simulink model "simSLIPModel"  (R2015a)
settings: Solver=ode45  StartTime=0.0  StopTime=2  FixedStep=0.001  RelTol=1e-6
values from neighbouring files (symbols this model uses):
  kIn = 50    [exhaustive.m]    (also in funkyFunc.m; heightConstraint.m; simVis.m)
  qIn = [q(1); q(2); dti; dri]    [exhaustive.m]    (also in funkyFunc.m; heightConstraint.m; simVis.m = [Thf0(1); Thf0(2); dti; dri])
  r0 = sym('r0', [noLinks 1])    [Generalised_SLIP_Model.m]    (also in Generalised_SLIP_Model_flight.m; exhaustive.m = 2; exhaustiveSearch.m = 2; funkyFunc.m = 2)
undefined symbols (not defined in the file or in its folder): k1, k2, k3, k4, k5
libraries: simulink x3, dspsigops x1
settings Model: Creator=STNNEI001  LastModifiedBy=STNNEI001
settings SolverCC: ZeroCrossAlgorithm=Adaptive
settings DataIOCC: ExternalInput=[qIn]  ReturnWorkspaceOutputs=on
settings DebuggingCC: UnderspecifiedInitializationDetection=Classic  MergeDetectMultiDrivingBlocksExec=none  MaxConsecutiveZCsMsg=none  MaskedZcDiagnostic=none  SolverPrmCheckMsg=warning  StateNameClashWarn=warning

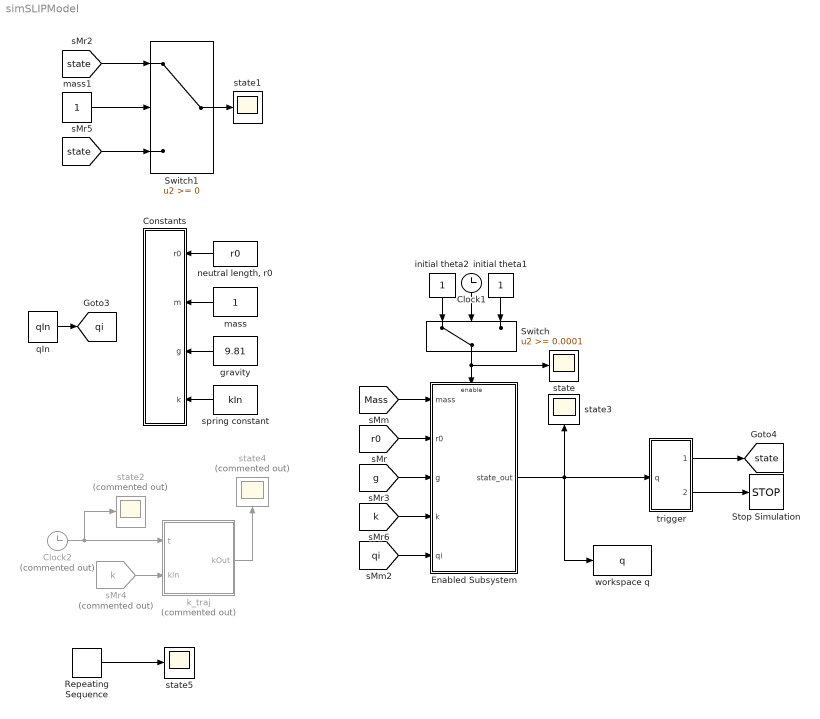
== system simSLIPModel ==
  Clock1 : Clock
  Clock2 : Clock  Commented=on
  Constants : Subsystem
  Enabled Subsystem : Subsystem  TreatAsAtomicUnit=on
  Repeating Sequence : simulink/Sources/Repeating Sequence  rep_seq_t=[0 0.05 0.1 0.15 0.32]  rep_seq_y=[k1 k2 k3 k4 k5]
  Stop Simulation : Stop
  Switch : Switch  Threshold=0.0001
  Switch1 : Switch
  gravity : Constant  Value=9.81
  initial theta1 : Constant
  initial theta2 : Constant
  k_traj : MATLAB Function  Commented=on  TreatAsAtomicUnit=on
  mass : Constant
  mass1 : Constant
  "neutral length, r0" : Constant  Value=r0
  qIn : Constant  Value=qIn
  sMr4 : From  Commented=on  GotoTag=k  TagVisibility=global
  spring constant : Constant  Value=kIn  VectorParams1D=off
  state{,1,3,5} (4 alike) : Scope
      state settings: SaveName=ScopeData16
      state1 settings: SaveName=ScopeData3
      state3 settings: SaveName=ScopeData15
      state5 settings: SaveName=ScopeData12
  state2 : Scope  Commented=on
      settings: SaveName=ScopeData4
  state4 : Scope  Commented=on
      settings: SaveName=ScopeData5
  trigger : Subsystem
  workspace q : ToWorkspace  VariableName=q  SaveFormat=Structure With Time  SampleTime=0.01
  tag scope: qi=global, state=global
  wires:
  "neutral length, r0"/1 -> Constants/1(r0)
  mass/1 -> Constants/2(m)
  gravity/1 -> Constants/3(g)
  spring constant/1 -> Constants/4(k)
  [Mass] -> Enabled Subsystem/1(mass)
  [r0] -> Enabled Subsystem/2(r0)
  [g] -> Enabled Subsystem/3(g)
  [qi] -> Enabled Subsystem/5(qi)
  Switch/1 -> state/1, Enabled Subsystem/Enable
  trigger/1(state) -> [state]
  Clock1/1 -> Switch/2
  initial theta1/1 -> Switch/3
  initial theta2/1 -> Switch/1
  Enabled Subsystem/1(state_out) -> trigger/1(q), workspace q/1, state3/1
  Switch1/1 -> state1/1
  [state] -> Switch1/1
  qIn/1 -> [qi]
  [state] -> Switch1/3
  sMr4/1 -> k_traj/2(kIn)
  Clock2/1 -> state2/1, k_traj/1(t)
  k_traj/1(kOut) -> state4/1
  [k] -> Enabled Subsystem/4(k)
  trigger/2(stop) -> Stop Simulation/1
  mass1/1 -> Switch1/2
  Repeating Sequence/1 -> state5/1

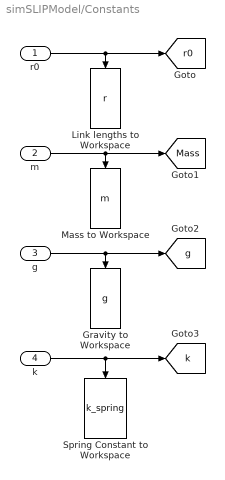
== system simSLIPModel/Constants ==
  r0 : Inport
  m : Inport  Port=2
  g : Inport  Port=3
  k : Inport  Port=4
  Gravity to Workspace : ToWorkspace  VariableName=g  SampleTime=-1
      settings: MaxDataPoints=1
  Link lengths to Workspace : ToWorkspace  VariableName=r  SampleTime=-1
      settings: MaxDataPoints=1
  Mass to Workspace : ToWorkspace  VariableName=m  SampleTime=-1
      settings: MaxDataPoints=1
  Spring Constant to Workspace : ToWorkspace  VariableName=k_spring  SampleTime=-1
      settings: MaxDataPoints=1
  tag scope: Mass=global, g=global, k=global, r0=global
  wires:
  m/1 -> [Mass], Mass to Workspace/1
  r0/1 -> Link lengths to Workspace/1, [r0]
  g/1 -> [g], Gravity to Workspace/1
  k/1 -> [k], Spring Constant to Workspace/1

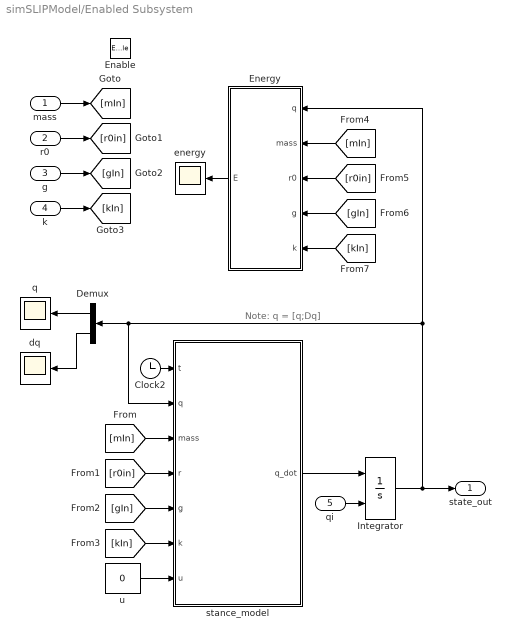
== system simSLIPModel/Enabled Subsystem ==
  note: Note: q = [q;Dq]
  mass : Inport
  r0 : Inport  Port=2
  g : Inport  Port=3
  k : Inport  Port=4
  qi : Inport  Port=5
  Enable : EnablePort
  Clock2 : Clock
  Demux : Demux  Outputs=2
  "Energy " : MATLAB Function  TreatAsAtomicUnit=on
  Integrator : Integrator  InitialConditionSource=external  InitialCondition=[pi/2;1;0;0]
  dq : Scope
      settings: SaveName=ScopeData7
  energy : Scope
  q : Scope
      settings: SaveName=ScopeData6
  stance_model : MATLAB Function  TreatAsAtomicUnit=on
  u : Constant  Value=0
  state_out : Outport
  wires:
  stance_model/1(q_dot) -> Integrator/1
  Integrator/1 -> state_out/1, stance_model/2(q), Demux/1, "Energy "/1(q)
  Demux/1 -> q/1
  Demux/2 -> dq/1
  [r0in] -> stance_model/4(r)
  [mIn] -> stance_model/3(mass)
  [gIn] -> stance_model/5(g)
  [kIn] -> stance_model/6(k)
  "Energy "/1(E) -> energy/1
  qi/1 -> Integrator/2
  u/1 -> stance_model/7(u)
  k/1 -> [kIn]
  g/1 -> [gIn]
  r0/1 -> [r0in]
  mass/1 -> [mIn]
  [mIn] -> "Energy "/2(mass)
  [r0in] -> "Energy "/3(r0)
  [gIn] -> "Energy "/4(g)
  [kIn] -> "Energy "/5(k)
  Clock2/1 -> stance_model/1(t)

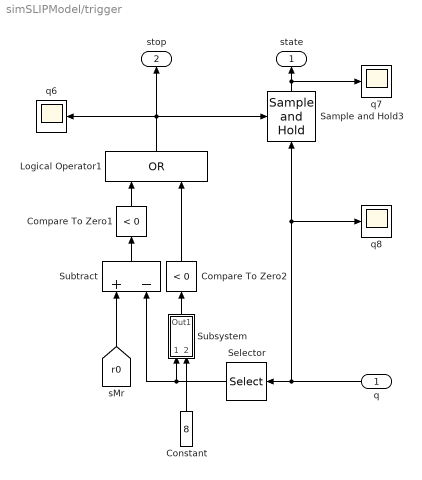
== system simSLIPModel/trigger ==
  q : Inport
  Compare To Zero1 : simulink/Logic and Bit Operations/Compare To Zero  relop=<  OutDataTypeStr=boolean
  Compare To Zero2 : simulink/Logic and Bit Operations/Compare To Zero  relop=<  OutDataTypeStr=boolean
  Constant : Constant  Value=8
  Logical Operator1 : Logic  Operator=OR  AllPortsSameDT=off  OutDataTypeStr=boolean
  Sample and Hold3 : dspsigops/Sample and Hold  trig=Rising edge  initCond=0  latchinput=off
  Selector : Selector  InputPortWidth=4  IndexOptions=Starting index (dialog)  Indices=[2]
  Subsystem : Subsystem
  Subtract : Sum  Inputs=+-
  q6 : Scope
      settings: SaveName=ScopeData2
  q7 : Scope
      settings: SaveName=ScopeData8
  q8 : Scope
      settings: SaveName=ScopeData11
  state : Outport
  stop : Outport  Port=2
  wires:
  Compare To Zero2/1 -> Logical Operator1/2
  Compare To Zero1/1 -> Logical Operator1/1
  Subtract/1 -> Compare To Zero1/1
  Logical Operator1/1 -> q6/1, Sample and Hold3/Trigger, stop/1
  q/1 -> Selector/1, q8/1, Sample and Hold3/1
  [r0] -> Subtract/1
  Sample and Hold3/1 -> q7/1, state/1
  Selector/1 -> Subtract/2, Subsystem/1(In1)
  Subsystem/1(Out1) -> Compare To Zero2/1
  Constant/1 -> Subsystem/2(In2)

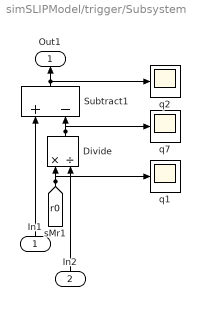
== system simSLIPModel/trigger/Subsystem ==
  In1 : Inport
  In2 : Inport  Port=2
  Divide : Product  Inputs=*/
  Subtract1 : Sum  Inputs=+-
  q1 : Scope
      settings: SaveName=ScopeData9
  q2 : Scope
      settings: SaveName=ScopeData10
  q7 : Scope
  Out1 : Outport
  wires:
  Divide/1 -> q7/1, Subtract1/2
  [r0] -> q1/1, Divide/1
  In1/1 -> Subtract1/1
  Subtract1/1 -> q2/1, Out1/1
  In2/1 -> Divide/2

== matlab function simSLIPModel/Enabled Subsystem/Energy  ==
  data: q input; E output; mass input; r0 input; g input; k input
function E = findEnergy(q,mass,r0,g,k)
%#codegen

    E = getEnergy(q,mass,r0,g,k);
end

== matlab function simSLIPModel/Enabled Subsystem/stance_model ==
  data: t input; q input; mass input; r input; g input; k input; u input; q_dot output
function q_dot  = simulinkModel(t,q,mass,r,g,k,u)
    %double_pen2 returns D2angle of the double pendulum with uniform mass
    %   Detailed explanation goes here
    n = size(q);
    n = n(1)/2;
    q_dot = zeros(2*n,1);
    q_dot(1:n) = q(n+1:2*n);
    q_dot(n+1:2*n) = ddq_func(q,mass,r,g,k,u);
end

== matlab function simSLIPModel/k_traj ==
  data: t input; kOut output; kIn input
function kOut = kTraj(t,kIn)
%#codegen
tTot = 5;
div = size(kIn,1)-1;
frac = t*(div/tTot);
i = floor(frac)+1;
i = min(i,div);
kOut = kIn(i)+(kIn(i+1)-kIn(i))*(frac+1-i);%[i;frac];
